simulink model "TORFPA_v4"  (R2022b)
settings: Solver=FixedStepAuto  StartTime=0.0  StopTime=0.04  FixedStep=1e-8  RelTol=1e-3
InitFcn:
  | Pole_pairs =2;
  | alphaOne= 0.59724;
  | alphaTwo = 0.92835;
  | alphaThree = 0.25059;;
  | Wo = 5000;
  | a0 = alphaOne;
  | a1 = alphaOne*Wo;
  | a2 = alphaTwo*Wo*Wo;
  | a3 = alphaThree*Wo*Wo*Wo;
  | dampening = 3;
undefined symbols (not defined in the file): DiscIntNeverNeededParam
libraries: simulink x3, dsparch4 x1
settings Model: Creator=e36916  LastModifiedBy=jarmusch

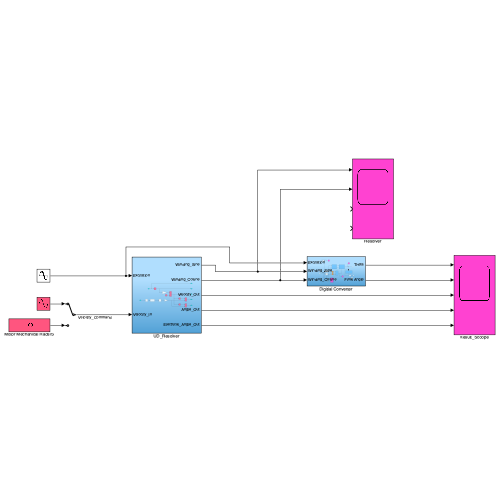
[thumbnail: Simulink's stored preview of the top-level diagram]
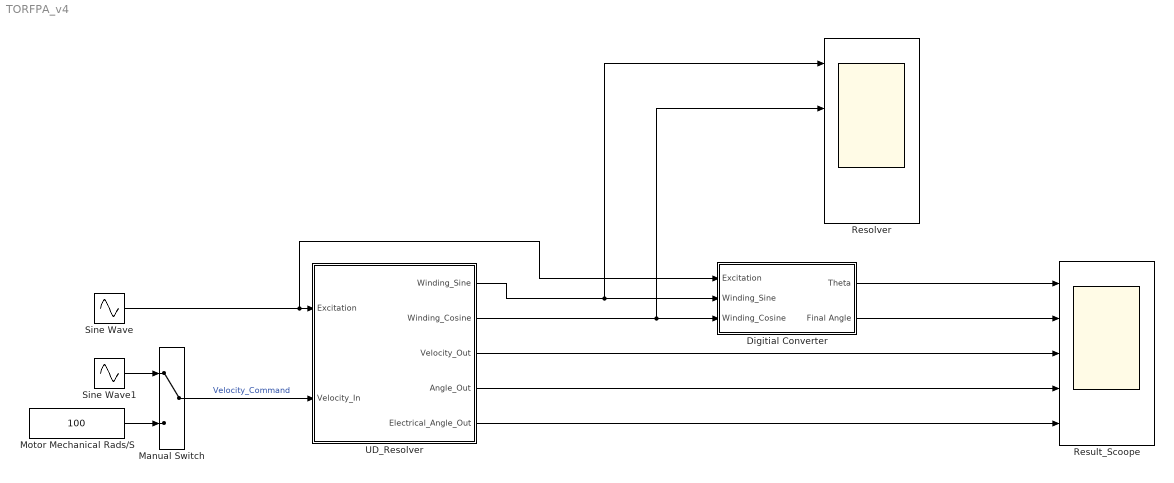
== system TORFPA_v4 ==
  Digitial Converter : Subsystem
  Manual Switch : ManualSwitch
  Motor Mechanical Rads/S : Constant  Value=100
  Resolver : Scope  NumInputPorts=4
  Result_Scoope : Scope  NumInputPorts=5
  Sine Wave : Sin  Amplitude=1.36  Bias=1.36  Frequency=2*pi*10000
  Sine Wave1 : Sin  Amplitude=3000  Frequency=50*pi  SampleTime=0
  UD_Resolver : Subsystem
  wires:
  Sine Wave1/1 -> Manual Switch/1
  Manual Switch/1 -> UD_Resolver/2(Velocity_In)  "Velocity_Command"
  Motor Mechanical Rads/S/1 -> Manual Switch/2
  UD_Resolver/3(Velocity_Out) -> Result_Scoope/3
  UD_Resolver/4(Angle_Out) -> Result_Scoope/4
  UD_Resolver/5(Electrical_Angle_Out) -> Result_Scoope/5
  UD_Resolver/1(Winding_Sine) -> Digitial Converter/2(Winding_Sine), Resolver/1
  UD_Resolver/2(Winding_Cosine) -> Digitial Converter/3(Winding_Cosine), Resolver/2
  Sine Wave/1 -> Digitial Converter/1(Excitation), UD_Resolver/1(Excitation)
  Digitial Converter/1(Theta) -> Result_Scoope/1
  Digitial Converter/2(Final Angle) -> Result_Scoope/2

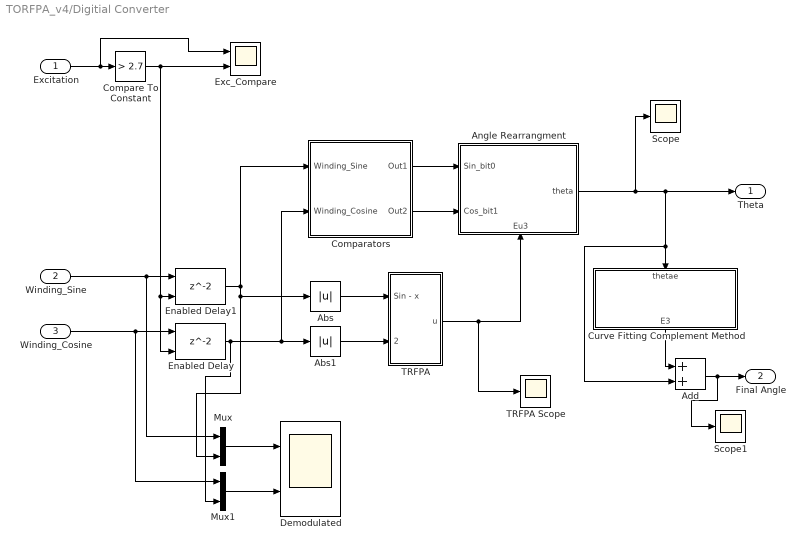
== system TORFPA_v4/Digitial Converter ==
  Excitation : Inport
  Winding_Sine : Inport  Port=2
  Winding_Cosine : Inport  Port=3
  Abs : Abs  SaturateOnIntegerOverflow=off
  Abs1 : Abs  SaturateOnIntegerOverflow=off
  Add : Sum
  Angle Rearrangment : Subsystem
      settings: PortSchema="{\"entries\":[{\"content\":{\"sides\":[{\"content\":{\"connectorIds\":[\"In1\",\"In2\"]},\"type\":\"ConnectorPlacement.EquallySpacedRectSide\",\"uuid\":\"c3e8efe3-e0ea-4274-93bd-3afae694db51\"},{\"content\":{\"connectorIds\":[\"Out1\"],\"side\":\"RIGHT\"},\"type\":\"ConnectorPlacement.EquallySpacedRectSide\",\"uuid\":\"d292ab8c-7c93-41a0-ab23-217f8069ff65\"},{\"content\":{\"connectorIds\":[],\"side\":\"TOP\"},\"type\":\"ConnectorPlacement.EquallySpacedRectSide\",\"uuid\":\"641c7881-a126-4f51-b37f-bbf9bf2de060\"},{\"content\":{\"connectorIds\":[\"In3\"],\"side\":\"BOTTOM\"},\"type\":\"ConnectorPlacement.EquallySpacedRectSide\",\"uuid\":\"c2284628-98df-446e-8c6d-cf576f2ccd66\"}]},\"type\":\"ConnectorPlacement.EquallySpacedConnector\",\"uuid\":\"91ec52a7-cd37-4479-8fd1-1be91748d98f\"}],\"packageUris\":[\"http://schema.mathworks.com/mf0/Connector/R2020b\"],\"version\":\"1.0\"}"
  Comparators : Subsystem
  Compare To Constant : simulink/Logic and Bit Operations/Compare To Constant  relop=>  const=2.7  OutDataTypeStr=boolean
  Curve Fitting Complement Method : Subsystem
      settings: PortSchema="{\"entries\":[{\"content\":{\"sides\":[{\"content\":{\"connectorIds\":[]},\"type\":\"ConnectorPlacement.EquallySpacedRectSide\",\"uuid\":\"72b05056-4a68-42b8-bec3-33582bdc67f7\"},{\"content\":{\"connectorIds\":[],\"side\":\"RIGHT\"},\"type\":\"ConnectorPlacement.EquallySpacedRectSide\",\"uuid\":\"48623c3b-a693-4a37-b1c5-dec080f838b8\"},{\"content\":{\"connectorIds\":[\"In1\"],\"side\":\"TOP\"},\"type\":\"ConnectorPlacement.EquallySpacedRectSide\",\"uuid\":\"529e6972-2e08-45e9-a571-f81a858e51f1\"},{\"content\":{\"connectorIds\":[\"Out1\"],\"side\":\"BOTTOM\"},\"type\":\"ConnectorPlacement.EquallySpacedRectSide\",\"uuid\":\"8a584edb-7ec7-4385-af1b-8d15923b4e6e\"}]},\"type\":\"ConnectorPlacement.EquallySpacedConnector\",\"uuid\":\"3a32fe3e-0c93-4aaa-9d65-7c8fc6bad786\"}],\"packageUris\":[\"http://schema.mathworks.com/mf0/Connector/R2020b\"],\"version\":\"1.0\"}"
  Demodulated : Scope  NumInputPorts=2
  Enabled Delay : Delay  ShowEnablePort=on
      settings: InputPortMap=u0,e6
  Enabled Delay1 : Delay  ShowEnablePort=on
      settings: InputPortMap=u0,e6
  Exc_Compare : Scope  NumInputPorts=2
  Mux : Mux  Inputs=2
  Mux1 : Mux  Inputs=2
  Scope : Scope
  Scope1 : Scope
  TRFPA : Subsystem
  TRFPA Scope : Scope
  Theta : Outport
  Final Angle : Outport  Port=2
  wires:
  Abs/1 -> TRFPA/1(Sin - x)
  Abs1/1 -> TRFPA/2(Cos - y)
  Comparators/1(Out1) -> Angle Rearrangment/1(Sin_bit0)
  Comparators/2(Out2) -> Angle Rearrangment/2(Cos_bit1)
  Angle Rearrangment/1(theta) -> Scope/1, Add/2, Curve Fitting Complement Method/1(thetae), Theta/1
  Curve Fitting Complement Method/1(E3) -> Add/1
  Add/1 -> Scope1/1, Final Angle/1
  TRFPA/1(u) -> TRFPA Scope/1, Angle Rearrangment/3(Eu3)
  Excitation/1 -> Exc_Compare/1, Compare To Constant/1
  Winding_Sine/1 -> Mux/1, Enabled Delay1/1
  Enabled Delay1/1 -> Mux/2, Abs/1, Comparators/1(Winding_Sine)
  Compare To Constant/1 -> Enabled Delay/2, Enabled Delay1/2, Exc_Compare/2
  Winding_Cosine/1 -> Enabled Delay/1, Mux1/1
  Enabled Delay/1 -> Mux1/2, Comparators/2(Winding_Cosine), Abs1/1
  Mux/1 -> Demodulated/1
  Mux1/1 -> Demodulated/2

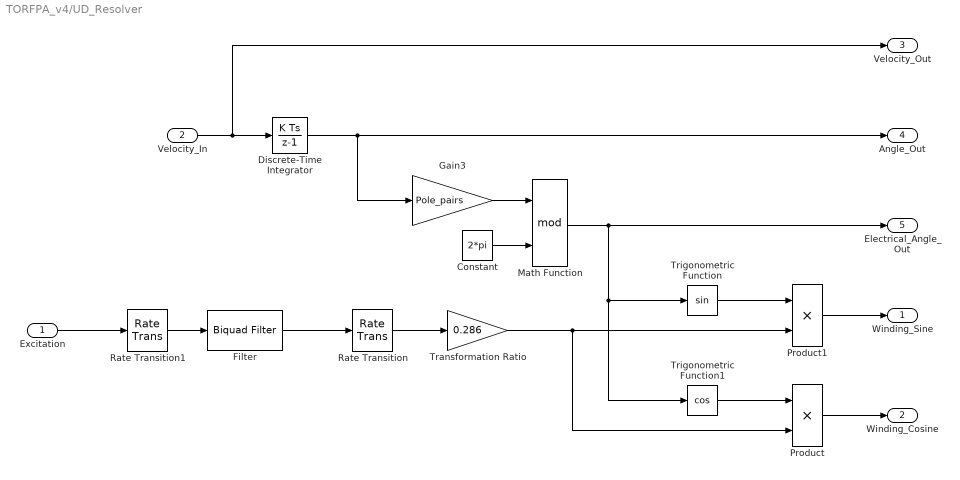
== system TORFPA_v4/UD_Resolver ==
  Excitation : Inport
  Velocity_In : Inport  Port=2
  Constant : Constant  Value=2*pi
  Discrete-Time Integrator : DiscreteIntegrator  SampleTime=-1  ICPrevOutput=DiscIntNeverNeededParam  ICPrevScaledInput=DiscIntNeverNeededParam
  Filter : dsparch4/Biquad Filter  Tag=BlockMethodSubSystem  FilterSource=Dialog parameters  CoeffSource=Specify via dialog  FilterObject=BQF  IIRFiltStruct=Direct form II  BiQuadCoeffs=[1 -2 1 1 -1.98532458709362158 0.98567733794518908;1 -2 1 1 -1.96541950338359084 0.965768717516137798]  ScaleValues=[0.992750481259702666;0.982797055224932214;1]  IC=0  ICnum=0  ICden=0  a0Flag=Warning  optimizeScaleValues=on  ScaleValueMode=Specify via input port (g)  InputProcessing=Columns as channels (frame based)  roundingMode=Floor  overflowMode=off  scaleValueFracLength=14  denProdOutputFracLength=30  denAccumFracLength=30  secondMemoryFracLength=15
  Gain3 : Gain  Gain=Pole_pairs
  Math Function : Math  Operator=mod
  Product : Product
  Product1 : Product
  Rate Transition : RateTransition  OutPortSampleTime=1e-8
  Rate Transition1 : RateTransition  OutPortSampleTime=1/1000000
  Transformation Ratio : Gain  Gain=0.286
  Trigonometric Function : Trigonometry
  Trigonometric Function1 : Trigonometry  Operator=cos
  Winding_Sine : Outport  VectorParamsAs1DForOutWhenUnconnected=off
  Winding_Cosine : Outport  Port=2  VectorParamsAs1DForOutWhenUnconnected=off
  Velocity_Out : Outport  Port=3  VectorParamsAs1DForOutWhenUnconnected=off
  Angle_Out : Outport  Port=4  VectorParamsAs1DForOutWhenUnconnected=off
  Electrical_Angle_Out : Outport  Port=5  VectorParamsAs1DForOutWhenUnconnected=off
  wires:
  Velocity_In/1 -> Velocity_Out/1, Discrete-Time Integrator/1
  Product1/1 -> Winding_Sine/1
  Transformation Ratio/1 -> Product/2, Product1/2
  Product/1 -> Winding_Cosine/1
  Excitation/1 -> Rate Transition1/1
  Discrete-Time Integrator/1 -> Angle_Out/1, Gain3/1
  Constant/1 -> Math Function/2
  Math Function/1 -> Electrical_Angle_Out/1, Trigonometric Function/1, Trigonometric Function1/1
  Gain3/1 -> Math Function/1
  Trigonometric Function/1 -> Product1/1
  Trigonometric Function1/1 -> Product/1
  Rate Transition1/1 -> Filter/1
  Rate Transition/1 -> Transformation Ratio/1
  Filter/1 -> Rate Transition/1

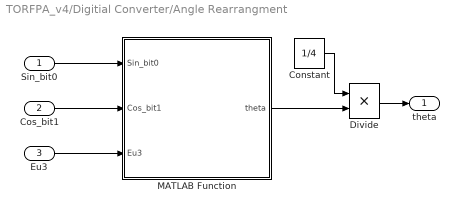
== system TORFPA_v4/Digitial Converter/Angle Rearrangment ==
  Sin_bit0 : Inport
  Cos_bit1 : Inport  Port=2
  Eu3 : Inport  Port=3
  Constant : Constant  Value=1/4
  Divide : Product  Inputs=**
  MATLAB Function : MATLAB Function  TreatAsAtomicUnit=on
  theta : Outport
  wires:
  Sin_bit0/1 -> MATLAB Function/1(Sin_bit0)
  Cos_bit1/1 -> MATLAB Function/2(Cos_bit1)
  Eu3/1 -> MATLAB Function/3(Eu3)
  MATLAB Function/1(theta) -> Divide/2
  Divide/1 -> theta/1
  Constant/1 -> Divide/1

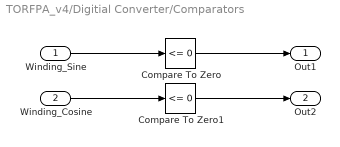
== system TORFPA_v4/Digitial Converter/Comparators ==
  Winding_Sine : Inport
  Winding_Cosine : Inport  Port=2
  Compare To Zero : simulink/Logic and Bit Operations/Compare To Zero  relop=<=  OutDataTypeStr=boolean
  Compare To Zero1 : simulink/Logic and Bit Operations/Compare To Zero  relop=<=  OutDataTypeStr=boolean
  Out1 : Outport
  Out2 : Outport  Port=2
  wires:
  Compare To Zero/1 -> Out1/1
  Winding_Sine/1 -> Compare To Zero/1
  Winding_Cosine/1 -> Compare To Zero1/1
  Compare To Zero1/1 -> Out2/1

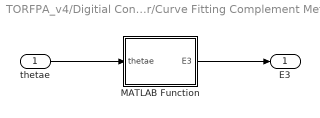
== system TORFPA_v4/Digitial Converter/Curve Fitting Complement Method ==
  thetae : Inport
  MATLAB Function : MATLAB Function  TreatAsAtomicUnit=on
  E3 : Outport
  wires:
  MATLAB Function/1(E3) -> E3/1
  thetae/1 -> MATLAB Function/1(thetae)

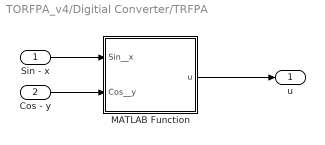
== system TORFPA_v4/Digitial Converter/TRFPA ==
  Sin - x : Inport
  Cos - y : Inport  Port=2
  MATLAB Function : MATLAB Function  TreatAsAtomicUnit=on
  u : Outport
  wires:
  Sin - x/1 -> MATLAB Function/1(Sin__x)
  Cos - y/1 -> MATLAB Function/2(Cos__y)
  MATLAB Function/1(u) -> u/1

== matlab function TORFPA_v4/Digitial Converter/Angle Rearrangment/MATLAB Function ==
  data: Sin_bit0 input; theta output; Cos_bit1 input; Eu3 input
function theta = fcn(Sin_bit0 , Cos_bit1, Eu3)

if ((Sin_bit0 == 0) && (Cos_bit1 == 0))
    theta = 0.25 * Eu3;
elseif ((Sin_bit0 == 0) && (Cos_bit1 == 1))
    theta = 0.5 - 0.25 * Eu3;
elseif ((Sin_bit0 == 1) && (Cos_bit1 == 1))
    theta = 0.5 + 0.25 * Eu3;
else %((Sin_bit0 == 1) && (Cos_bit1 == 0))
    theta = 1 - 0.25 * Eu3;
end

== matlab function TORFPA_v4/Digitial Converter/TRFPA/MATLAB Function ==
  data: Sin__x input; u output; Cos__y input
function u = fcn(Sin__x, Cos__y)

%u = (Cos__y/(Sin__x + Cos__y))*( ((0.64039 * Sin__x^2) + (Sin__x * Cos__y) + (Cos__y^2)) / ((Sin__x^2) + (0.64039*Sin__x*Cos__y) + (Cos__y^2)));
u = 1-(Cos__y/(Sin__x + Cos__y))*( ((0.64039 * Sin__x^2) + (Sin__x * Cos__y) + (Cos__y^2)) / ((Sin__x^2) + (0.64039*Sin__x*Cos__y) + (Cos__y^2)));

== matlab function TORFPA_v4/Digitial Converter/Curve Fitting Complement Method/MATLAB Function ==
  data: thetae input; E3 output
function E3 = fcn(thetae)

%E3 = (-20.2404*thetae + 111.2857*thetae - 239.6213*thetae + 254.4939*thetae - 137.1434*thetae + 33.9851*thetae - 2.7004*thetae - 0.0155) / 1000;
E3 = (-20.2404*thetae^7 + 111.2857*thetae^6 - 239.6213*thetae^5 + 254.4939*thetae^4 - 137.1434*thetae^3 + 33.9851*thetae^2 - 2.7004*thetae - 0.0155) / 1000;
